simulink model "sampleModel1678"  (R2023a)
settings: Solver=VariableStepAuto  StartTime=0.0  StopTime=10.0  RelTol=1e-3
libraries: hdlsllib x5, simulink x4
settings Model: Creator=user1  LastModifiedBy=user1

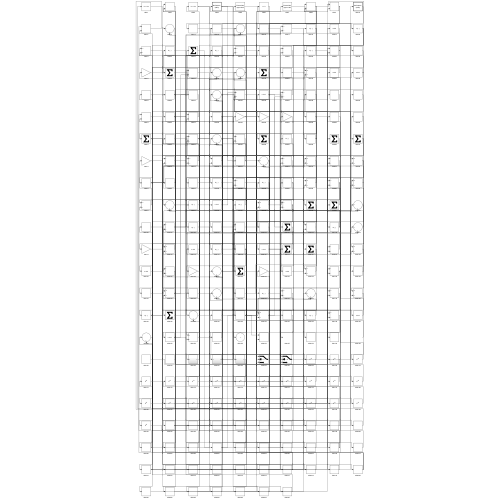
[thumbnail: Simulink's stored preview of the top-level diagram]
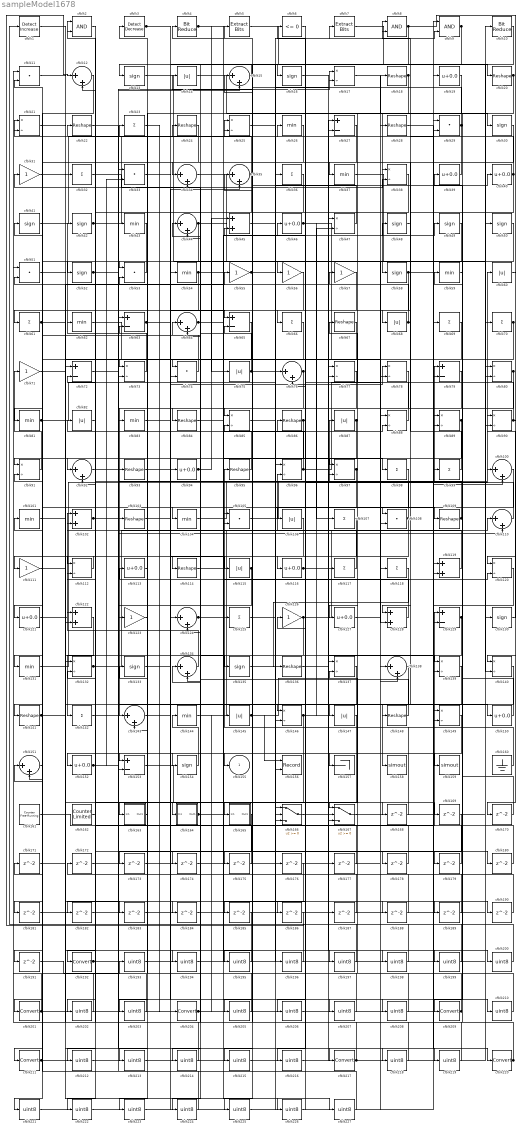
== system sampleModel1678 ==
  cfblk1 : simulink/Logic and Bit Operations/Detect Increase  vinit=0.0  OutDataTypeStr=boolean
      settings: LibrarySourceBlock=|
      | hdlsllib/Logic and Bit
      | Operations/Detect
      | Increase
  cfblk10 : hdlsllib/Logic and Bit Operations/Bit Reduce  mode=AND
  cfblk{12,15,34..35,44,64,76,92,100,110,124,134,138,143,151} (15 alike) : Sum  Inputs=|++
  cfblk{26,37,43,54,59,62,81,83,101,104,131,144} (12 alike) : MinMax
  cfblk{45,102,119,122,128} (5 alike) : Sum
  cfblk{18,20,22,24,28,67,84,86,93,95,103,109,114,136,141,148} (16 alike) : Reshape
  cfblk{11,29,33,51,53,74,105,108} (8 alike) : DotProduct  OutDataTypeStr=Inherit: Inherit via internal rule
  cfblk{14,60,68,75,82,87,106,115,145,147} (10 alike) : Abs  SaturateOnIntegerOverflow=off
  cfblk{23,32,36,61,66,69..70,98..99,107,117..118,125,142} (14 alike) : Sum  Inputs=+
  cfblk{31,55..57,71,111,123,126} (8 alike) : Gain
  cfblk{17,21,25,38,47,73,77..78,80,85,88..91,96..97,112,120,132,137,139..140,146,149} (24 alike) : Product  Inputs=*/  RndMeth=Zero  SaturateOnIntegerOverflow=on
  cfblk{19,39..40,46,94,113,116,121,127,150,152} (11 alike) : Bias  Bias=0.0  SaturateOnIntegerOverflow=off
  cfblk{27,63,65,72,79,129,153} (7 alike) : Sum  Inputs=+-
  cfblk{13,16,30,41..42,48..50,52,58,130,133,135,154} (14 alike) : Signum
  cfblk156 : Record  FileSettingsInternal="{\"entries\":[{\"content\":{\"excelSettings\":{\"content\":{},\"type\":\"Streamout.ExcelSettings\"}},\"type\":\"Streamout.FileSettingStorage\",\"uuid\":\"\"}],\"packageUris\":[\"http:\\/\\/schema.mathworks.com\\/mf0\\/streamout_blocks\\/R2020a\"],\"version\":\"1.0\"}"  Layout=[1 1]  SignalsInternal="{\"entries\":[{\"content\":{\"signals\":[{\"content\":{\"blockPath\":[],\"dimensions\":[1],\"domain\":\"\",\"lineColor\":\"#a2142f\",\"plots\":[1],\"port\":1,\"signalID\":2860,\"signalName\":\"XY Graph:1\"},\"type\":\"RecordBlkView.Signal\",\"uuid\":\"\"},{\"content\":{\"blockPath\":[],\"dimensions\":[1],\"domain\":\"\",\"lineColor\":\"#139fff\",\"plots\":[1],\"port\":2,\"signalID\":2863,\"signalName\":\"XY Graph:2\"},\"type\":\"RecordBlkView.Signal\",\"uuid\":\"\"}]},\"type\":\"RecordBlkView.InputSignals\",\"uuid\":\"\"}],\"packageUris\":[\"http:\\/\\/schema.mathworks.com\\/mf0\\/streamout_blocks\\/R2020a\"],\"version\":\"1.0\"}"  VisualizationBindings="{\"xyplotplugin\":{\"info\":[{\"series\":[{\"bindingParametersList\":[{\"parameter\":\"X-Axis\",\"signalID\":2860,\"signalName\":\"XY Graph:1\"},{\"parameter\":\"Y-Axis\",\"signalID\":2863,\"signalName\":\"XY Graph:2\"}],\"seriesID\":25122}],\"subplotID\":1}]}}"  CompatibilityTag=XY  st=-1
  cfblk157 : Terminator
  cfblk158 : ToWorkspace  VariableName=simout  SaveFormat=Timeseries  SampleTime=-1
  cfblk159 : ToWorkspace  VariableName=simout  SaveFormat=Timeseries  SampleTime=-1
  cfblk160 : Ground
  cfblk161 : hdlsllib/Sources/Counter Free-Running  NumBits=16  tsamp=-1
  cfblk162 : hdlsllib/Sources/Counter Limited  uplimit=7  tsamp=-1
  cfblk163 : Subsystem
      settings: LibrarySourceBlock=|
      | hdlsllib/Ports &
      | Subsystems/Subsystem
  cfblk164 : Subsystem
      settings: LibrarySourceBlock=|
      | hdlsllib/Ports &
      | Subsystems/Subsystem
  cfblk165 : Subsystem
      settings: LibrarySourceBlock=|
      | hdlsllib/Ports &
      | Subsystems/Subsystem
  cfblk166 : Switch  SaturateOnIntegerOverflow=off  InputSameDT=off
  cfblk167 : Switch  SaturateOnIntegerOverflow=off  InputSameDT=off
  cfblk{168..191} (24 alike) : Delay  SampleTime=1
  cfblk{192,201,204,209,211,217,220} (7 alike) : DataTypeConversion  SaturateOnIntegerOverflow=off  RndMeth=Floor
  cfblk{193..200,202..203,205..208,210,212..216,218..219,221..227} (29 alike) : DataTypeConversion  OutDataTypeStr=uint8  SaturateOnIntegerOverflow=off  RndMeth=Floor
  cfblk2 : Logic  AllPortsSameDT=off  OutDataTypeStr=boolean
  cfblk3 : simulink/Logic and Bit Operations/Detect Decrease  vinit=0.0  OutDataTypeStr=boolean
      settings: LibrarySourceBlock=|
      | hdlsllib/Logic and Bit
      | Operations/Detect
      | Decrease
  cfblk4 : hdlsllib/Logic and Bit Operations/Bit Reduce  mode=AND
  cfblk5 : simulink/Logic and Bit Operations/Extract Bits  bitsToExtract=Upper half  numBits=8  bitIdxRange=[0 7]  outScalingMode=Preserve fixed-point scaling
      settings: LibrarySourceBlock=|
      | hdlsllib/Logic and Bit
      | Operations/Extract Bits
  cfblk6 : hdlsllib/Logic and Bit Operations/Compare To Zero  relop=<=  OutDataTypeStr=boolean
  cfblk7 : simulink/Logic and Bit Operations/Extract Bits  bitsToExtract=Upper half  numBits=8  bitIdxRange=[0 7]  outScalingMode=Preserve fixed-point scaling
      settings: LibrarySourceBlock=|
      | hdlsllib/Logic and Bit
      | Operations/Extract Bits
  cfblk8 : Logic  AllPortsSameDT=off  OutDataTypeStr=boolean
  cfblk9 : Logic  AllPortsSameDT=off  OutDataTypeStr=boolean
  cfblk155 : Outport  VectorParamsAs1DForOutWhenUnconnected=off
  wires:
  cfblk34/1 -> cfblk56/1
  cfblk19/1 -> cfblk58/1
  cfblk35/1 -> cfblk22/1, cfblk73/2
  cfblk9/1 -> cfblk92/1, cfblk156/2
  cfblk28/1 -> cfblk220/1
  cfblk93/1 -> cfblk94/1
  cfblk131/1 -> cfblk60/1
  cfblk134/1 -> cfblk102/1
  cfblk105/1 -> cfblk79/1
  cfblk70/1 -> cfblk73/1, cfblk141/1
  cfblk48/1 -> cfblk128/1
  cfblk8/1 -> cfblk140/1, cfblk34/1, cfblk216/1
  cfblk118/1 -> cfblk136/1
  cfblk67/1 -> cfblk163/1(In1)
  cfblk161/1 -> cfblk129/1
  cfblk108/1 -> cfblk21/2, cfblk186/1
  cfblk5/1 -> cfblk20/1
  cfblk52/1 -> cfblk26/1, cfblk178/1
  cfblk23/1 -> cfblk204/1
  cfblk87/1 -> cfblk143/1, cfblk127/1
  cfblk38/1 -> cfblk104/1
  cfblk15/1 -> cfblk13/1
  cfblk96/1 -> cfblk18/1, cfblk44/2
  cfblk141/1 -> cfblk147/1, cfblk183/1
  cfblk36/1 -> cfblk192/1
  cfblk86/1 -> cfblk116/1, cfblk131/1, cfblk124/2
  cfblk55/1 -> cfblk109/1, cfblk167/3
  cfblk56/1 -> cfblk112/1
  cfblk75/1 -> cfblk31/1, cfblk78/2
  cfblk39/1 -> cfblk37/1
  cfblk160/1 -> cfblk95/1
  cfblk99/1 -> cfblk8/1
  cfblk42/1 -> cfblk25/1, cfblk24/1
  cfblk31/1 -> cfblk25/2
  cfblk148/1 -> cfblk64/1
  cfblk91/1 -> cfblk71/1
  cfblk59/1 -> cfblk209/1
  cfblk12/1 -> cfblk81/1
  cfblk77/1 -> cfblk85/1
  cfblk71/1 -> cfblk165/1(In1)
  cfblk125/1 -> cfblk17/1
  cfblk14/1 -> cfblk70/1
  cfblk76/1 -> cfblk103/1, cfblk213/1
  cfblk83/1 -> cfblk54/1
  cfblk22/1 -> cfblk93/1
  cfblk104/1 -> cfblk87/1
  cfblk113/1 -> cfblk143/2
  cfblk80/1 -> cfblk84/1, cfblk225/1
  cfblk37/1 -> cfblk130/1
  cfblk151/1 -> cfblk201/1
  cfblk41/1 -> cfblk19/1
  cfblk29/1 -> cfblk4/1, cfblk68/1
  cfblk126/1 -> cfblk110/1, cfblk174/1
  cfblk27/1 -> cfblk211/1
  cfblk13/1 -> cfblk80/1
  cfblk127/1 -> cfblk49/1
  cfblk154/1 -> cfblk144/1
  cfblk64/1 -> cfblk134/2, cfblk189/1, cfblk190/1
  cfblk130/1 -> cfblk90/1
  cfblk140/1 -> cfblk158/1
  cfblk132/1 -> cfblk77/2, cfblk33/2
  cfblk163/1(Out1) -> cfblk3/1
  cfblk21/1 -> cfblk32/1
  cfblk95/1 -> cfblk2/1
  cfblk94/1 -> cfblk44/1, cfblk45/1
  cfblk122/1 -> cfblk142/1
  cfblk144/1 -> cfblk9/1
  cfblk149/1 -> cfblk152/1
  cfblk73/1 -> cfblk42/1
  cfblk128/1 -> cfblk113/1
  cfblk51/1 -> cfblk217/1
  cfblk7/1 -> cfblk140/2
  cfblk11/1 -> cfblk135/1
  cfblk47/1 -> cfblk14/1
  cfblk119/1 -> cfblk12/2
  cfblk103/1 -> cfblk149/2
  cfblk62/1 -> cfblk166/1
  cfblk146/1 -> cfblk47/2, cfblk182/1, cfblk200/1
  cfblk117/1 -> cfblk46/1
  cfblk123/1 -> cfblk63/2
  cfblk82/1 -> cfblk62/1
  cfblk115/1 -> cfblk175/1, cfblk223/1
  cfblk150/1 -> cfblk39/1
  cfblk79/1 -> cfblk119/2
  cfblk135/1 -> cfblk9/2
  cfblk124/1 -> cfblk96/2, cfblk48/1
  cfblk17/1 -> cfblk30/1
  cfblk40/1 -> cfblk148/1, cfblk8/2
  cfblk74/1 -> cfblk21/1
  cfblk167/1 -> cfblk90/2
  cfblk20/1 -> cfblk123/1, cfblk167/1, cfblk159/1
  cfblk4/1 -> cfblk125/1, cfblk167/2, cfblk75/1
  cfblk112/1 -> cfblk111/1
  cfblk2/1 -> cfblk92/2
  cfblk129/1 -> cfblk155/1, cfblk89/2
  cfblk92/1 -> cfblk110/2
  cfblk109/1 -> cfblk5/1, cfblk82/1
  cfblk153/1 -> cfblk166/2
  cfblk142/1 -> cfblk17/2
  cfblk26/1 -> cfblk114/1
  cfblk18/1 -> cfblk164/1(In1), cfblk97/1
  cfblk89/1 -> cfblk153/1, cfblk91/1
  cfblk98/1 -> cfblk157/1
  cfblk61/1 -> cfblk74/1, cfblk150/1
  cfblk46/1 -> cfblk128/2, cfblk107/1
  cfblk121/1 -> cfblk122/1
  cfblk54/1 -> cfblk98/1, cfblk146/1, cfblk181/1
  cfblk6/1 -> cfblk66/1
  cfblk97/1 -> cfblk166/3, cfblk221/1
  cfblk24/1 -> cfblk61/1
  cfblk66/1 -> cfblk122/2
  cfblk120/1 -> cfblk129/2
  cfblk114/1 -> cfblk76/1
  cfblk88/1 -> cfblk67/1
  cfblk68/1 -> cfblk57/1, cfblk41/1, cfblk108/1
  cfblk143/1 -> cfblk78/1
  cfblk3/1 -> cfblk16/1, cfblk65/1
  cfblk116/1 -> cfblk139/1, cfblk168/1
  cfblk164/1(Out1) -> cfblk88/2, cfblk120/2
  cfblk90/1 -> cfblk120/1, cfblk45/2
  cfblk145/1 -> cfblk117/1, cfblk156/1, cfblk47/1, cfblk188/1
  cfblk152/1 -> cfblk43/1, cfblk208/1
  cfblk111/1 -> cfblk55/1
  cfblk57/1 -> cfblk83/1
  cfblk110/1 -> cfblk6/1
  cfblk63/1 -> cfblk115/1, cfblk35/2
  cfblk44/1 -> cfblk118/1, cfblk53/1, cfblk89/1
  cfblk53/1 -> cfblk52/1
  cfblk30/1 -> cfblk38/1
  cfblk139/1 -> cfblk153/2
  cfblk58/1 -> cfblk106/1, cfblk100/2
  cfblk106/1 -> cfblk121/1
  cfblk81/1 -> cfblk40/1, cfblk7/1, cfblk33/1
  cfblk65/1 -> cfblk154/1
  cfblk102/1 -> cfblk15/2, cfblk100/1
  cfblk162/1 -> cfblk2/2
  cfblk32/1 -> cfblk38/2
  cfblk168/1 -> cfblk15/1
  cfblk166/1 -> cfblk169/1
  cfblk60/1 -> cfblk170/1
  cfblk170/1 -> cfblk79/2
  cfblk49/1 -> cfblk173/1
  cfblk173/1 -> cfblk88/1
  cfblk174/1 -> cfblk97/2
  cfblk175/1 -> cfblk102/2
  cfblk136/1 -> cfblk177/1
  cfblk177/1 -> cfblk112/2
  cfblk178/1 -> cfblk134/1
  cfblk45/1 -> cfblk179/1
  cfblk179/1 -> cfblk96/1
  cfblk25/1 -> cfblk180/1
  cfblk180/1 -> cfblk35/1
  cfblk181/1 -> cfblk80/2
  cfblk182/1 -> cfblk119/1
  cfblk183/1 -> cfblk149/1
  cfblk147/1 -> cfblk184/1
  cfblk100/1 -> cfblk185/1
  cfblk185/1 -> cfblk1/1
  cfblk186/1 -> cfblk12/1
  cfblk187/1 -> cfblk77/1
  cfblk188/1 -> cfblk76/2
  cfblk189/1 -> cfblk132/2
  cfblk190/1 -> cfblk85/2
  cfblk50/1 -> cfblk191/1
  cfblk192/1 -> cfblk108/2, cfblk124/1, cfblk50/1
  cfblk191/1 -> cfblk193/1
  cfblk193/1 -> cfblk36/1
  cfblk72/1 -> cfblk194/1
  cfblk194/1 -> cfblk105/2
  cfblk169/1 -> cfblk195/1
  cfblk195/1 -> cfblk72/1
  cfblk85/1 -> cfblk196/1
  cfblk196/1 -> cfblk72/2
  cfblk171/1 -> cfblk197/1
  cfblk197/1 -> cfblk105/1
  cfblk16/1 -> cfblk198/1
  cfblk198/1 -> cfblk171/1
  cfblk133/1 -> cfblk199/1
  cfblk199/1 -> cfblk11/2
  cfblk200/1 -> cfblk133/1
  cfblk201/1 -> cfblk74/2, cfblk11/1
  cfblk165/1(Out1) -> cfblk202/1
  cfblk202/1 -> cfblk151/1
  cfblk107/1 -> cfblk203/1
  cfblk203/1 -> cfblk151/2
  cfblk204/1 -> cfblk187/1, cfblk145/1
  cfblk10/1 -> cfblk205/1
  cfblk205/1 -> cfblk23/1
  cfblk137/1 -> cfblk206/1
  cfblk206/1 -> cfblk29/2
  cfblk184/1 -> cfblk207/1
  cfblk207/1 -> cfblk137/1
  cfblk208/1 -> cfblk137/2
  cfblk209/1 -> cfblk53/2, cfblk29/1
  cfblk33/1 -> cfblk210/1
  cfblk210/1 -> cfblk59/1
  cfblk211/1 -> cfblk139/2, cfblk146/2, cfblk91/2, cfblk10/1
  cfblk43/1 -> cfblk212/1
  cfblk212/1 -> cfblk27/1
  cfblk213/1 -> cfblk27/2
  cfblk138/1 -> cfblk214/1
  cfblk214/1 -> cfblk172/1
  cfblk78/1 -> cfblk215/1
  cfblk215/1 -> cfblk138/1
  cfblk216/1 -> cfblk138/2
  cfblk217/1 -> cfblk64/2, cfblk132/1
  cfblk1/1 -> cfblk218/1
  cfblk218/1 -> cfblk51/1
  cfblk172/1 -> cfblk219/1
  cfblk219/1 -> cfblk51/2
  cfblk220/1 -> cfblk65/2, cfblk99/1, cfblk126/1
  cfblk221/1 -> cfblk28/1
  cfblk176/1 -> cfblk222/1
  cfblk222/1 -> cfblk34/2
  cfblk223/1 -> cfblk176/1
  cfblk69/1 -> cfblk224/1
  cfblk224/1 -> cfblk63/1
  cfblk225/1 -> cfblk69/1
  cfblk101/1 -> cfblk226/1
  cfblk226/1 -> cfblk86/1
  cfblk84/1 -> cfblk227/1
  cfblk227/1 -> cfblk101/1

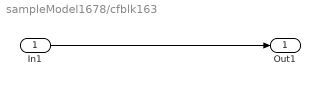
== system sampleModel1678/cfblk163 ==
  In1 : Inport
  Out1 : Outport
  wires:
  In1/1 -> Out1/1

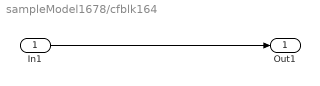
== system sampleModel1678/cfblk164 ==
  In1 : Inport
  Out1 : Outport
  wires:
  In1/1 -> Out1/1

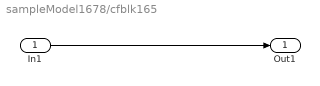
== system sampleModel1678/cfblk165 ==
  In1 : Inport
  Out1 : Outport
  wires:
  In1/1 -> Out1/1
